simulink model "BDRSOn"  (R2018b)
settings: Solver=FixedStepAuto  StartTime=0.0  StopTime=10.0  RelTol=1e-3
libraries: simulink x5
settings Model: DataDictionary=Master_Dictionary.sldd  Creator=torni  LastModifiedBy=Build
settings RTWCC: SystemTargetFile=erpt_grt.tlc  TemplateMakefile=erpt_grt_default_tmf  Description=ETAS Rapid Prototyping Target
settings STFCustomTargetCC: TargetLangStandard=C99 (ISO)  UtilityFuncGeneration=Shared location  GRTInterface=on  SystemTargetFile=erpt_grt.tlc
settings GRTTargetCC: UtilityFuncGeneration=Shared location  ParMdlRefBuildCompliant=off  CompOptLevelCompliant=off  ConcurrentExecutionCompliant=off  CombineOutputUpdateFcns=off  MatFileLogging=off  CPPClassGenCompliant=off  GRTInterface=on  UseToolchainInfoCompliant=off  GenerateASAP2=on

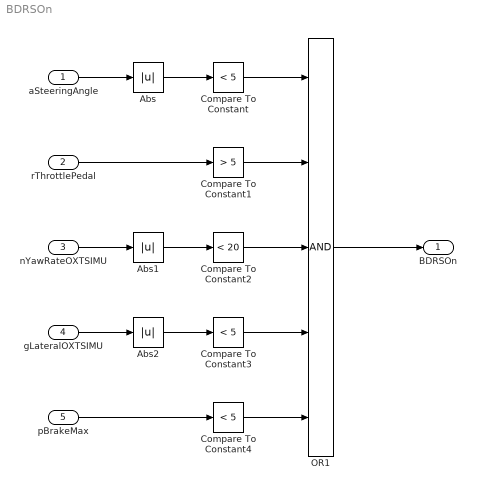
== system BDRSOn ==
  aSteeringAngle : Inport  OutDataTypeStr=double
  rThrottlePedal : Inport  Port=2  OutDataTypeStr=double
  nYawRateOXTSIMU : Inport  Port=3  OutDataTypeStr=double
  gLateralOXTSIMU : Inport  Port=4  OutDataTypeStr=double
  pBrakeMax : Inport  Port=5  OutDataTypeStr=double
  Abs : Abs
  Abs1 : Abs
  Abs2 : Abs
  Compare To Constant : simulink/Logic and Bit Operations/Compare To Constant  relop=<  const=5  OutDataTypeStr=boolean
  Compare To Constant1 : simulink/Logic and Bit Operations/Compare To Constant  relop=>  const=5  OutDataTypeStr=boolean
  Compare To Constant2 : simulink/Logic and Bit Operations/Compare To Constant  relop=<  const=20  OutDataTypeStr=boolean
  Compare To Constant3 : simulink/Logic and Bit Operations/Compare To Constant  relop=<  const=5  OutDataTypeStr=boolean
  Compare To Constant4 : simulink/Logic and Bit Operations/Compare To Constant  relop=<  const=5  OutDataTypeStr=boolean
  OR1 : Logic  Inputs=5  AllPortsSameDT=off  OutDataTypeStr=boolean
  BDRSOn : Outport  OutDataTypeStr=boolean
  wires:
  OR1/1 -> BDRSOn/1
  aSteeringAngle/1 -> Abs/1
  rThrottlePedal/1 -> Compare To Constant1/1
  nYawRateOXTSIMU/1 -> Abs1/1
  gLateralOXTSIMU/1 -> Abs2/1
  pBrakeMax/1 -> Compare To Constant4/1
  Compare To Constant/1 -> OR1/1
  Compare To Constant1/1 -> OR1/2
  Compare To Constant2/1 -> OR1/3
  Abs/1 -> Compare To Constant/1
  Abs1/1 -> Compare To Constant2/1
  Abs2/1 -> Compare To Constant3/1
  Compare To Constant3/1 -> OR1/4
  Compare To Constant4/1 -> OR1/5
